simulink model "rx_channelizer_PL"  (R2024a)
settings: Solver=VariableStepAuto  StartTime=0.0  StopTime=num_ch*150/fs  RelTol=1e-3
PreLoadFcn:
  | ch_rate = 41e6; % per channel sample rate
  | num_ch = 32;
  | flip_cnt = num_ch/2 - 1; % flip data count size
  | % 6 coeffs/ch;
  | PLclk=ch_rate*16; % PL clock frequency
  | fs = ch_rate*num_ch;
  | sample_rate = 1/fs;
  | base_freq=1e6; % what base channel frequency to modulate?
  | 
  | generate_prototype_FIR; % create FIR coeffs
undefined symbols (not defined in the file): ch0, ch1, ch10, ch11, ch12, ch13, ch14, ch15, ch16, ch17, ch18, ch19, ch2, ch20, ch21, ch22, ch23, ch24, ch25, ch26, ch27, ch28, ch29, ch3, ch30, ch31, ch4, ch5, ch6, ch7, ch8, ch9, S, vsva2197, xcvc1902
libraries: hdlBasic x69, dspsrcs4 x4, hdlSSR x3, hdlDSPIP x2, dspmlti4 x1, dspxfrm3 x1, vmcUtilities x1
(part 2 of 2)

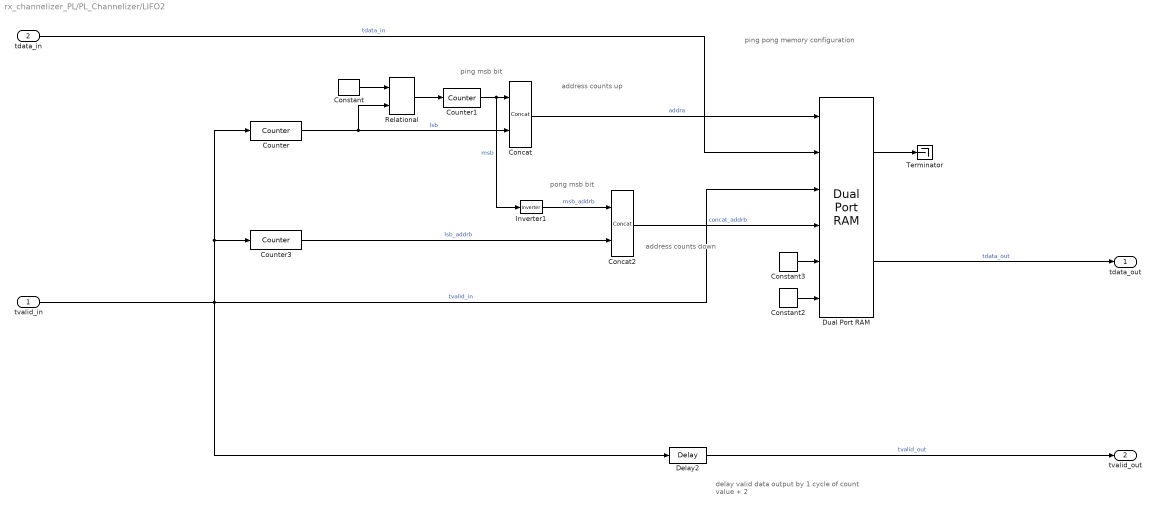
== system rx_channelizer_PL/PL_Channelizer/LIFO2 ==
  note: pong msb bit
  note: address counts down
  note: ping pong memory configuration
  note: address counts up
  note: ping msb bit
  note: delay valid data output by 1 cycle of count value + 2
  tvalid_in : Inport
  tdata_in : Inport  Port=2
  Concat : hdlBasic/Concat  num_inputs=2  XmcBlockStatus=1  maskContainerNames=group1  block_type=concat  block_config=sysgen:Concat_config
  Concat2 : hdlBasic/Concat  num_inputs=2  XmcBlockStatus=1  maskContainerNames=group1  block_type=concat  block_config=sysgen:Concat_config
  Constant : hdlBasic/Constant  const=flip_cnt  gui_display_data_type=Fixed-point  arith_type=Unsigned  n_bits=ceil(log2(flip_cnt))  bin_pt=0  preci_type=Single  exp_width=8  frac_width=24  explicit_period=off  period=1  XmcBlockStatus=1  maskContainerNames=tabcontainer1  block_type=constant  block_config=sysgen:Constant_config
  Constant2 : hdlBasic/Constant  const=0  gui_display_data_type=Boolean  arith_type=Boolean  n_bits=16  bin_pt=14  preci_type=Single  exp_width=8  frac_width=24  explicit_period=off  period=1  XmcBlockStatus=1  maskContainerNames=tabcontainer1  block_type=constant  block_config=sysgen:Constant_config
  Constant3 : hdlBasic/Constant  const=0  gui_display_data_type=Fixed-point  arith_type=Unsigned  n_bits=23  bin_pt=22  preci_type=Single  exp_width=8  frac_width=24  explicit_period=off  period=1  XmcBlockStatus=1  maskContainerNames=tabcontainer1  block_type=constant  block_config=sysgen:Constant_config
  Counter : hdlBasic/Counter  cnt_type=Count limited  cnt_to=flip_cnt  operation=Up  start_count=0  cnt_by_val=1  arith_type=Unsigned  n_bits=ceil(log2(flip_cnt))  bin_pt=0  load_pin=off  rst=off  en=on  explicit_period=Inferred from inputs  period=1  use_behavioral_HDL=off  implementation=Fabric  XmcBlockStatus=1  maskContainerNames=group1  block_type=counter  block_config=sysgen:Counter_config  block_width=531  block_height=1023
  Counter1 : hdlBasic/Counter  cnt_type=Free running  cnt_to=Inf  operation=Up  start_count=0  cnt_by_val=1  arith_type=Unsigned  n_bits=1  bin_pt=0  load_pin=off  rst=off  en=on  explicit_period=Inferred from inputs  period=1  use_behavioral_HDL=off  implementation=Fabric  XmcBlockStatus=1  maskContainerNames=group1  block_type=counter  block_config=sysgen:Counter_config  block_width=531  block_height=1023
  Counter3 : hdlBasic/Counter  cnt_type=Count limited  cnt_to=0  operation=Down  start_count=flip_cnt  cnt_by_val=1  arith_type=Unsigned  n_bits=ceil(log2(flip_cnt))  bin_pt=0  load_pin=off  rst=off  en=on  explicit_period=Inferred from inputs  period=1  use_behavioral_HDL=off  implementation=Fabric  XmcBlockStatus=1  maskContainerNames=group1  block_type=counter  block_config=sysgen:Counter_config  block_width=531  block_height=1023
  Delay2 : hdlBasic/Delay  rst=off  en=off  latency=flip_cnt+2  reg_retiming=off  XmcBlockStatus=1  maskContainerNames=group1  block_type=delay  block_config=sysgen:Delay_config
  Dual Port RAM : hdlBasic/Dual Port RAM  depth=2^(ceil(log2(flip_cnt)+1))  initVector=zeros(2^(ceil(log2(flip_cnt)+1)))  distributed_mem=Block RAM  init_a=0  init_b=0  rst_a=off  rst_b=off  en_a=off  en_b=off  latency=1  write_mode_A=Read After Write  write_mode_B=Read After Write  explicit_period=[]  period=[]  simulation_type=fast_sim  XmcBlockStatus=1  maskContainerNames=tabcontainer1  block_type=dpram  block_config=sysgen:Dpram_config  optimize=Area
      settings: infoedit=[]
  Inverter1 : hdlBasic/Inverter  en=off  latency=0  XmcBlockStatus=1  maskContainerNames=group2  block_type=inv  block_config=sysgen:Inverter_config
  Relational : hdlBasic/Relational  mode=a=b  op_type=Bool  en=off  latency=0  XmcBlockStatus=1  maskContainerNames=tabcontainer1  block_type=relational  block_config=sysgen:Relational_config
  Terminator : Terminator
  tdata_out : Outport
  tvalid_out : Outport  Port=2
  wires:
  tdata_in/1 -> Dual Port RAM/2  "tdata_in"
  Concat2/1 -> Dual Port RAM/4  "concat_addrb"
  Counter3/1 -> Concat2/2  "lsb_addrb"
  Inverter1/1 -> Concat2/1  "msb_addrb"
  Counter1/1 -> Concat/1, Inverter1/1  "msb"
  Dual Port RAM/1 -> Terminator/1
  tvalid_in/1 -> Delay2/1, Dual Port RAM/3, Counter/1, Counter3/1  "tvalid_in"
  Dual Port RAM/2 -> tdata_out/1  "tdata_out"
  Constant/1 -> Relational/1
  Delay2/1 -> tvalid_out/1  "tvalid_out"
  Counter/1 -> Concat/2, Relational/2  "lsb"
  Concat/1 -> Dual Port RAM/1  "addra"
  Constant2/1 -> Dual Port RAM/6
  Relational/1 -> Counter1/1
  Constant3/1 -> Dual Port RAM/5

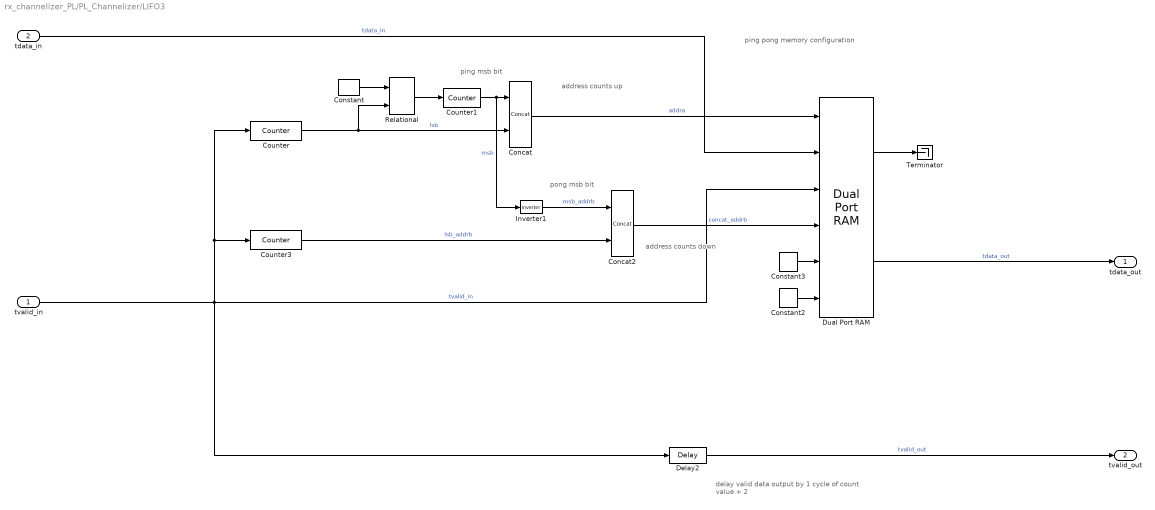
== system rx_channelizer_PL/PL_Channelizer/LIFO3 ==
  note: delay valid data output by 1 cycle of count value + 2
  note: ping msb bit
  note: address counts up
  note: ping pong memory configuration
  note: address counts down
  note: pong msb bit
  tvalid_in : Inport
  tdata_in : Inport  Port=2
  Concat : hdlBasic/Concat  num_inputs=2  XmcBlockStatus=1  maskContainerNames=group1  block_type=concat  block_config=sysgen:Concat_config
  Concat2 : hdlBasic/Concat  num_inputs=2  XmcBlockStatus=1  maskContainerNames=group1  block_type=concat  block_config=sysgen:Concat_config
  Constant : hdlBasic/Constant  const=flip_cnt  gui_display_data_type=Fixed-point  arith_type=Unsigned  n_bits=ceil(log2(flip_cnt))  bin_pt=0  preci_type=Single  exp_width=8  frac_width=24  explicit_period=off  period=1  XmcBlockStatus=1  maskContainerNames=tabcontainer1  block_type=constant  block_config=sysgen:Constant_config
  Constant2 : hdlBasic/Constant  const=0  gui_display_data_type=Boolean  arith_type=Boolean  n_bits=16  bin_pt=14  preci_type=Single  exp_width=8  frac_width=24  explicit_period=off  period=1  XmcBlockStatus=1  maskContainerNames=tabcontainer1  block_type=constant  block_config=sysgen:Constant_config
  Constant3 : hdlBasic/Constant  const=0  gui_display_data_type=Fixed-point  arith_type=Unsigned  n_bits=23  bin_pt=22  preci_type=Single  exp_width=8  frac_width=24  explicit_period=off  period=1  XmcBlockStatus=1  maskContainerNames=tabcontainer1  block_type=constant  block_config=sysgen:Constant_config
  Counter : hdlBasic/Counter  cnt_type=Count limited  cnt_to=flip_cnt  operation=Up  start_count=0  cnt_by_val=1  arith_type=Unsigned  n_bits=ceil(log2(flip_cnt))  bin_pt=0  load_pin=off  rst=off  en=on  explicit_period=Inferred from inputs  period=1  use_behavioral_HDL=off  implementation=Fabric  XmcBlockStatus=1  maskContainerNames=group1  block_type=counter  block_config=sysgen:Counter_config  block_width=531  block_height=1023
  Counter1 : hdlBasic/Counter  cnt_type=Free running  cnt_to=Inf  operation=Up  start_count=0  cnt_by_val=1  arith_type=Unsigned  n_bits=1  bin_pt=0  load_pin=off  rst=off  en=on  explicit_period=Inferred from inputs  period=1  use_behavioral_HDL=off  implementation=Fabric  XmcBlockStatus=1  maskContainerNames=group1  block_type=counter  block_config=sysgen:Counter_config  block_width=531  block_height=1023
  Counter3 : hdlBasic/Counter  cnt_type=Count limited  cnt_to=0  operation=Down  start_count=flip_cnt  cnt_by_val=1  arith_type=Unsigned  n_bits=ceil(log2(flip_cnt))  bin_pt=0  load_pin=off  rst=off  en=on  explicit_period=Inferred from inputs  period=1  use_behavioral_HDL=off  implementation=Fabric  XmcBlockStatus=1  maskContainerNames=group1  block_type=counter  block_config=sysgen:Counter_config  block_width=531  block_height=1023
  Delay2 : hdlBasic/Delay  rst=off  en=off  latency=flip_cnt+2  reg_retiming=off  XmcBlockStatus=1  maskContainerNames=group1  block_type=delay  block_config=sysgen:Delay_config
  Dual Port RAM : hdlBasic/Dual Port RAM  depth=2^(ceil(log2(flip_cnt)+1))  initVector=zeros(2^(ceil(log2(flip_cnt)+1)))  distributed_mem=Block RAM  init_a=0  init_b=0  rst_a=off  rst_b=off  en_a=off  en_b=off  latency=1  write_mode_A=Read After Write  write_mode_B=Read After Write  explicit_period=[]  period=[]  simulation_type=fast_sim  XmcBlockStatus=1  maskContainerNames=tabcontainer1  block_type=dpram  block_config=sysgen:Dpram_config  optimize=Area
      settings: infoedit=[]
  Inverter1 : hdlBasic/Inverter  en=off  latency=0  XmcBlockStatus=1  maskContainerNames=group2  block_type=inv  block_config=sysgen:Inverter_config
  Relational : hdlBasic/Relational  mode=a=b  op_type=Bool  en=off  latency=0  XmcBlockStatus=1  maskContainerNames=tabcontainer1  block_type=relational  block_config=sysgen:Relational_config
  Terminator : Terminator
  tdata_out : Outport
  tvalid_out : Outport  Port=2
  wires:
  Constant3/1 -> Dual Port RAM/5
  Relational/1 -> Counter1/1
  Constant2/1 -> Dual Port RAM/6
  Concat/1 -> Dual Port RAM/1  "addra"
  Counter/1 -> Relational/2, Concat/2  "lsb"
  Delay2/1 -> tvalid_out/1  "tvalid_out"
  Constant/1 -> Relational/1
  Dual Port RAM/2 -> tdata_out/1  "tdata_out"
  tvalid_in/1 -> Counter3/1, Counter/1, Dual Port RAM/3, Delay2/1  "tvalid_in"
  Dual Port RAM/1 -> Terminator/1
  Counter1/1 -> Inverter1/1, Concat/1  "msb"
  Inverter1/1 -> Concat2/1  "msb_addrb"
  Counter3/1 -> Concat2/2  "lsb_addrb"
  Concat2/1 -> Dual Port RAM/4  "concat_addrb"
  tdata_in/1 -> Dual Port RAM/2  "tdata_in"

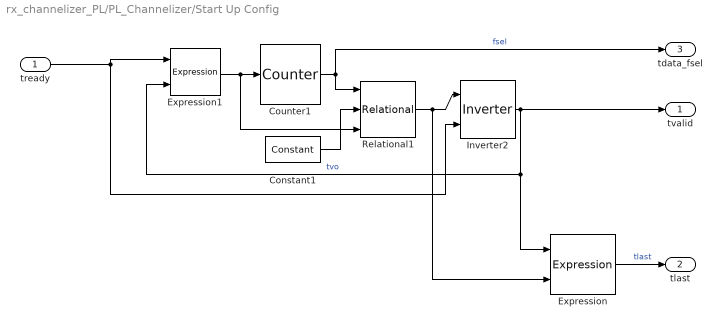
== system rx_channelizer_PL/PL_Channelizer/Start Up Config ==
  tready : Inport
  Constant1 : hdlBasic/Constant  const=14  gui_display_data_type=Fixed-point  arith_type=Unsigned  n_bits=4  bin_pt=0  preci_type=Single  exp_width=8  frac_width=24  explicit_period=off  period=1  XmcBlockStatus=1  maskContainerNames=tabcontainer1  block_type=constant  block_config=sysgen:Constant_config
  Counter1 : hdlBasic/Counter  cnt_type=Free running  cnt_to=Inf  operation=Up  start_count=0  cnt_by_val=1  arith_type=Unsigned  n_bits=4  bin_pt=0  load_pin=off  rst=off  en=on  explicit_period=Explicit  period=1/PLclk  use_behavioral_HDL=off  implementation=Fabric  XmcBlockStatus=1  maskContainerNames=group1  block_type=counter  block_config=sysgen:Counter_config  block_width=531  block_height=1023
  Expression : hdlBasic/Expression  expression=a & b  align_bp=on  en=off  latency=0  precision=Full  arith_type=Unsigned  n_bits=16  bin_pt=0  XmcBlockStatus=1  maskContainerNames=tabcontainer1  block_type=expr  block_config=sysgen:Expr_config
  Expression1 : hdlBasic/Expression  expression=a & b  align_bp=on  en=off  latency=0  precision=Full  arith_type=Unsigned  n_bits=16  bin_pt=0  XmcBlockStatus=1  maskContainerNames=tabcontainer1  block_type=expr  block_config=sysgen:Expr_config
  Inverter2 : hdlBasic/Inverter  en=on  latency=1  XmcBlockStatus=1  maskContainerNames=group2  block_type=inv  block_config=sysgen:Inverter_config
  Relational1 : hdlBasic/Relational  mode=a>=b  op_type=Bool  en=on  latency=1  XmcBlockStatus=1  maskContainerNames=tabcontainer1  block_type=relational  block_config=sysgen:Relational_config
  tvalid : Outport
  tlast : Outport  Port=2
  tdata_fsel : Outport  Port=3
  wires:
  Inverter2/1 -> Expression1/2, Expression/1, tvalid/1  "tvo"
  tready/1 -> Expression1/1, Inverter2/2
  Counter1/1 -> Relational1/1, tdata_fsel/1  "fsel"
  Constant1/1 -> Relational1/2
  Relational1/1 -> Expression/2, Inverter2/1
  Expression1/1 -> Counter1/1, Relational1/3
  Expression/1 -> tlast/1  "tlast"
